simulink model "Three_Voltmeter_method"  (R2021a)
settings: Solver=VariableStepAuto  StartTime=0.0  StopTime=0.05  RelTol=1e-3
libraries: spsRMSLib x4, spsVoltageMeasurementLib x3, spsCurrentMeasurementLib x2, spsSeriesRLCBranchLib x2, spsACVoltageSourceLib x1, spsGroundLib x1, spsPowerLib x1, spspowerguiLib x1
settings Model: Creator=tuhin  LastModifiedBy=sayan

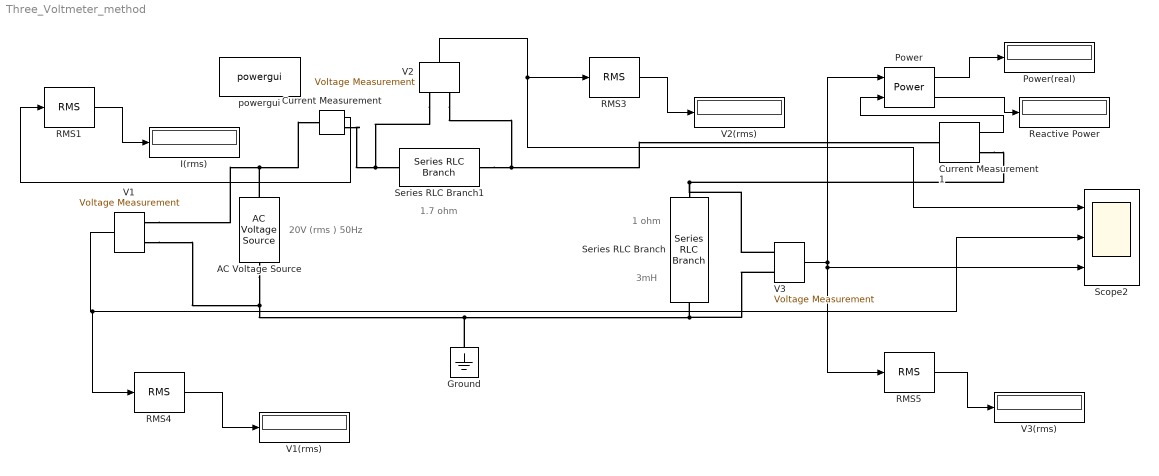
== system Three_Voltmeter_method ==
  note: 20V (rms )
      | 50Hz
  note: 3mH
  note: 1 ohm
  note: 1.7 ohm
  AC Voltage Source : spsACVoltageSourceLib/AC Voltage Source  Amplitude=28.28427125  Phase=0  Frequency=50  SampleTime=1e-6  Measurements=Voltage  BusType=swing  Pref=10e3  Qref=0  Qmin=-inf  Qmax=+inf
  Current Measurement : spsCurrentMeasurementLib/Current Measurement  PhasorSimulation=off  OutputType=Complex  PSBequivalent=0
  Current Measurement1 : spsCurrentMeasurementLib/Current Measurement  PhasorSimulation=off  OutputType=Complex  PSBequivalent=0
  Ground : spsGroundLib/Ground  LConnTagsString=a
  I(rms) : Display
  Power : spsPowerLib/Power  Freq=60  Vinit=[1, 0]  Iinit=[1, 0]  Ts=0
      settings: SourceProductBaseCode=PS
  Power(real) : Display
  RMS{1,3..5} (4 alike) : spsRMSLib/RMS  TrueRMS=on  Freq=50  RMSInit=0  Ts=0
  Reactive Power : Display
  Scope2 : Scope  NumInputPorts=3
  Series RLC Branch : spsSeriesRLCBranchLib/Series RLC Branch  LConnTagsString=__new0  RConnTagsString=__new0  BranchType=RL  Resistance=1  Inductance=3e-3  SetiL0=off  InitialCurrent=0  Capacitance=1e-6  Setx0=off  InitialVoltage=0  Measurements=None
  Series RLC Branch1 : spsSeriesRLCBranchLib/Series RLC Branch  LConnTagsString=__new0  RConnTagsString=__new0  BranchType=R  Resistance=1.7  Inductance=2e-3  SetiL0=off  InitialCurrent=0  Capacitance=1e-6  Setx0=off  InitialVoltage=0  Measurements=None
  V1 : spsVoltageMeasurementLib/Voltage Measurement  PhasorSimulation=off  OutputType=Complex  PSBequivalent=0
  V1(rms) : Display
  V2 : spsVoltageMeasurementLib/Voltage Measurement  PhasorSimulation=off  OutputType=Complex  PSBequivalent=0
  V2(rms) : Display
  V3 : spsVoltageMeasurementLib/Voltage Measurement  PhasorSimulation=off  OutputType=Complex  PSBequivalent=0
  V3(rms) : Display
  powergui : spspowerguiLib/powergui  Priority=1  SimulationMode=Continuous  SampleTime=50e-6  frequency=60  Iterations=50  frequencyindice=50  Pbase=100e6  ErrMax=1e-4  UnitsV=kV  UnitsW=MW  buscounter=0  FunctionMessages=off  echomessages=off  EnableUseOfTLC=off  CurrentSourceSwitches=off  DisableSnubberDevices=off  DisableRonSwitches=off  DisableVfSwitches=off  DisplayEquations=off  AutomaticDiscreteSolvers=off  SolverType=Tustin/Backward Euler (TBE)  Interpol=off  ExternalGateDelay=off  methode=off  Ts=100  x0status=blocks  SPID=on  SwTol=0  HookPort=off  NonlinearTolerance=1e-4  nMaxIteration=100  ContinueOnMaxIteration=off  RestoreLinks=warning  ResistiveCurrentMeasurement=off  Frange=[0:2:500]  Ylog=off  Xlog=on  ShowGrid=off  save=off  variable=ZData  structure=0  ZoomFFT=off  StartTime=0.0  cycles=1  DisplayStyle=1  fundamental=60  FreqAxis=off  MaxFrequency=1000  frequencyindicesteady=1  RmsSteady=1  display=off
  wires:
  V2/1 -> RMS3/1, Scope2/1
  V3/1 -> RMS5/1, Scope2/3, Power/1
  RMS5/1 -> V3(rms)/1
  V1/1 -> RMS4/1, Scope2/2
  RMS4/1 -> V1(rms)/1
  RMS3/1 -> V2(rms)/1
  RMS1/1 -> I(rms)/1
  Current Measurement/1 -> RMS1/1
  Current Measurement1/1 -> Power/2
  Power/1 -> Power(real)/1
  Power/2 -> Reactive Power/1
  connections:
  AC Voltage Source/RConn1 -- V1/LConn2 -- Current Measurement/LConn1
  Series RLC Branch1/RConn1 -- V2/LConn2 -- Current Measurement1/LConn1
  AC Voltage Source/LConn1 -- Ground/LConn1 -- V3/LConn2 -- Series RLC Branch/RConn1 -- V1/LConn1
  Current Measurement/RConn1 -- V2/LConn1 -- Series RLC Branch1/LConn1
  Current Measurement1/RConn1 -- V3/LConn1 -- Series RLC Branch/LConn1
